simulink model "Simulink_crane_hardware_model_SingleContr_R2016a"  (R2016a)
settings: Solver=ode5  StartTime=0.0  StopTime=inf  FixedStep=1/100  RelTol=1e-3  AbsTol=1e-6
values from neighbouring files (symbols this model uses):
  DTraj = 0.3    [RunHWModel.m]
  ITraj = 0.3    [RunHWModel.m]
  PTraj = 3.0    (= 3)    [RunHWModel.m]
  Ts = 1/20    (= 0.05)    [setup.m]
  waypoints = [waypoints, find_nearest_obstacles(waypoints, Grid)]    [path_planning.m]    (also in path_to_waypoints.m = [])
undefined symbols (not defined in the file or in its folder): Crane3D_RangeBit, Crane3D_ScaleCoeff, xRange, yRange
undefined symbols (not defined in the file): RTDAC4PCIBaseAddress
libraries: simulink x2
(part 11 of 11)

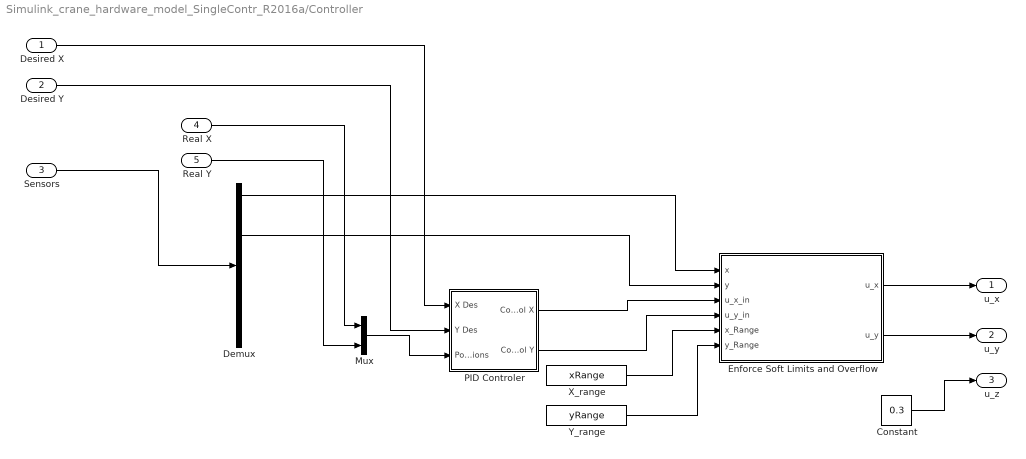
== system Simulink_crane_hardware_model_SingleContr_R2016a/Controller ==
  Desired X : Inport
  Desired Y : Inport  Port=2
  Sensors : Inport  Port=3
  Real X : Inport  Port=4
  Real Y : Inport  Port=5
  Constant : Constant  Value=0.3
  Demux : Demux  Outputs=8
  Enforce Soft Limits and Overflow : MATLAB Function  TreatAsAtomicUnit=on
      settings: PermitHierarchicalResolution=ParametersOnly
  Mux : Mux  Inputs=2
  PID Controler : Subsystem
  X_range : Constant  Value=xRange
  "Y_range " : Constant  Value=yRange
  u_x : Outport
  u_y : Outport  Port=2
  u_z : Outport  Port=3
  wires:
  Constant/1 -> u_z/1
  "Y_range "/1 -> Enforce Soft Limits and Overflow/6(y_Range)
  X_range/1 -> Enforce Soft Limits and Overflow/5(x_Range)
  PID Controler/2(Control Y) -> Enforce Soft Limits and Overflow/4(u_y_in)
  PID Controler/1(Control X) -> Enforce Soft Limits and Overflow/3(u_x_in)
  Desired X/1 -> PID Controler/1(X Des)
  Enforce Soft Limits and Overflow/2(u_y) -> u_y/1
  Enforce Soft Limits and Overflow/1(u_x) -> u_x/1
  Desired Y/1 -> PID Controler/2(Y Des)
  Mux/1 -> PID Controler/3(Positions)
  Sensors/1 -> Demux/1
  Demux/1 -> Enforce Soft Limits and Overflow/1(x)
  Demux/3 -> Enforce Soft Limits and Overflow/2(y)
  Real X/1 -> Mux/1
  Real Y/1 -> Mux/2

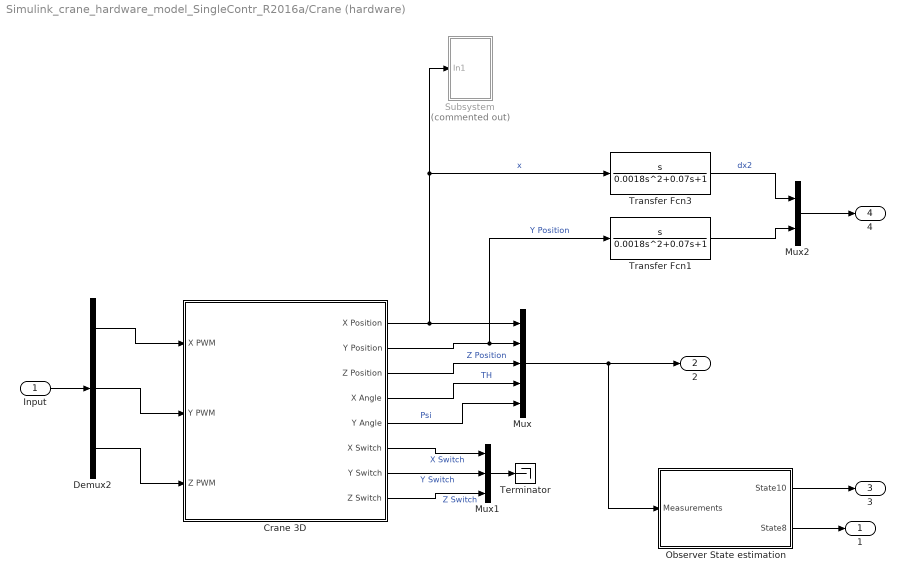
== system Simulink_crane_hardware_model_SingleContr_R2016a/Crane (hardware) ==
  Input : Inport
  Crane 3D : Subsystem  mask{BaseAddress=RTDAC4PCIBaseAddress, T0=1/100}
      mask prompts: BaseAddress "Base Address:"; T0 "Sampling Period:"
      mask Display: image(imread('crane.jpeg'))
  Demux2 : Demux  Outputs=3
  Mux : Mux  Inputs=5
  Mux1 : Mux  Inputs=3
  Mux2 : Mux  Inputs=2
  Observer State estimation : Subsystem
  Subsystem : Subsystem  Commented=on
  Terminator : Terminator
  Transfer Fcn1 : TransferFcn  Numerator=[1 0]  Denominator=[0.0018 0.07 1]
  Transfer Fcn3 : TransferFcn  Numerator=[1 0]  Denominator=[0.0018 0.07 1]
  1 : Outport
  2 : Outport  Port=2
  3 : Outport  Port=3
  4 : Outport  Port=4
  wires:
  Input/1 -> Demux2/1
  Crane 3D/2(Y Position) -> Transfer Fcn1/1, Mux/2  "Y Position"
  Crane 3D/3(Z Position) -> Mux/3  "Z Position"
  Crane 3D/4(X Angle) -> Mux/4  "TH"
  Crane 3D/5(Y Angle) -> Mux/5  "Psi"
  Mux/1 -> 2/1, Observer State estimation/1(Measurements)
  Crane 3D/6(X Switch) -> Mux1/1  "X Switch"
  Crane 3D/7(Y Switch) -> Mux1/2  "Y Switch"
  Crane 3D/8(Z Switch) -> Mux1/3  "Z Switch"
  Demux2/1 -> Crane 3D/1(X PWM)
  Demux2/2 -> Crane 3D/2(Y PWM)
  Demux2/3 -> Crane 3D/3(Z PWM)
  Observer State estimation/2(State8) -> 1/1
  Mux1/1 -> Terminator/1
  Observer State estimation/1(State10) -> 3/1
  Crane 3D/1(X Position) -> Subsystem/1(In1), Transfer Fcn3/1, Mux/1  "x"
  Transfer Fcn3/1 -> Mux2/1  "dx2"
  Transfer Fcn1/1 -> Mux2/2
  Mux2/1 -> 4/1

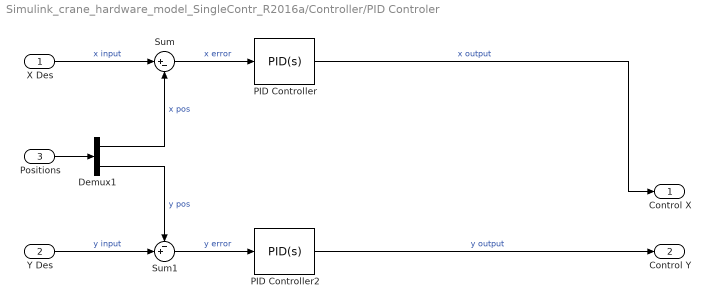
== system Simulink_crane_hardware_model_SingleContr_R2016a/Controller/PID Controler ==
  X Des : Inport
  Y Des : Inport  Port=2
  Positions : Inport  Port=3
  Demux1 : Demux  Outputs=2
  PID Controller : simulink/Continuous/PID Controller  Controller=PID  TimeDomain=Continuous-time  SampleTime=-1  IntegratorMethod=Forward Euler  FilterMethod=Forward Euler  Form=Parallel  UseFilter=on  ControllerParametersSource=internal  P=PTraj  I=ITraj  D=DTraj  N=30  InitialConditionSource=internal  InitialConditionForIntegrator=0  InitialConditionForFilter=0  ExternalReset=none  LimitOutput=on  UpperSaturationLimit=1  LowerSaturationLimit=-1  LinearizeAsGain=on  AntiWindupMode=none  Kb=1  TrackingMode=off  Kt=1  PParamMin=[]  PParamMax=[]  IParamMin=[]  IParamMax=[]  DParamMin=[]  DParamMax=[]  NParamMin=[]  NParamMax=[]  KbParamMin=[]  KbParamMax=[]  KtParamMin=[]  KtParamMax=[]  POutMin=[]  POutMax=[]  IOutMin=[]  IOutMax=[]  DOutMin=[]  DOutMax=[]  NOutMin=[]  NOutMax=[]  KbOutMin=[]  KbOutMax=[]  KtOutMin=[]  KtOutMax=[]  IntegratorOutMin=[]  IntegratorOutMax=[]  FilterOutMin=[]  FilterOutMax=[]  SumOutMin=[]  SumOutMax=[]  SumI1OutMin=[]  SumI1OutMax=[]  SumI2OutMin=[]  SumI2OutMax=[]  SumI3OutMin=[]  SumI3OutMax=[]  SumDOutMin=[]  SumDOutMax=[]  SaturationOutMin=[]  SaturationOutMax=[]  IntegratorContinuousStateAttributes=''  IntegratorStateMustResolveToSignalObject=off  IntegratorRTWStateStorageClass=Auto  FilterContinuousStateAttributes=''  FilterStateMustResolveToSignalObject=off  FilterRTWStateStorageClass=Auto  DifferentiatorICPrevScaledInput=0  DifferentiatorOutMin=[]  DifferentiatorOutMax=[]
  PID Controller2 : simulink/Continuous/PID Controller  Controller=PID  TimeDomain=Continuous-time  SampleTime=-1  IntegratorMethod=Forward Euler  FilterMethod=Forward Euler  Form=Parallel  UseFilter=on  ControllerParametersSource=internal  P=PTraj  I=ITraj  D=DTraj  N=30  InitialConditionSource=internal  InitialConditionForIntegrator=0  InitialConditionForFilter=0  ExternalReset=none  LimitOutput=on  UpperSaturationLimit=1  LowerSaturationLimit=-1  LinearizeAsGain=on  AntiWindupMode=none  Kb=1  TrackingMode=off  Kt=1  PParamMin=[]  PParamMax=[]  IParamMin=[]  IParamMax=[]  DParamMin=[]  DParamMax=[]  NParamMin=[]  NParamMax=[]  KbParamMin=[]  KbParamMax=[]  KtParamMin=[]  KtParamMax=[]  POutMin=[]  POutMax=[]  IOutMin=[]  IOutMax=[]  DOutMin=[]  DOutMax=[]  NOutMin=[]  NOutMax=[]  KbOutMin=[]  KbOutMax=[]  KtOutMin=[]  KtOutMax=[]  IntegratorOutMin=[]  IntegratorOutMax=[]  FilterOutMin=[]  FilterOutMax=[]  SumOutMin=[]  SumOutMax=[]  SumI1OutMin=[]  SumI1OutMax=[]  SumI2OutMin=[]  SumI2OutMax=[]  SumI3OutMin=[]  SumI3OutMax=[]  SumDOutMin=[]  SumDOutMax=[]  SaturationOutMin=[]  SaturationOutMax=[]  IntegratorContinuousStateAttributes=''  IntegratorStateMustResolveToSignalObject=off  IntegratorRTWStateStorageClass=Auto  FilterContinuousStateAttributes=''  FilterStateMustResolveToSignalObject=off  FilterRTWStateStorageClass=Auto  DifferentiatorICPrevScaledInput=0  DifferentiatorOutMin=[]  DifferentiatorOutMax=[]
  Sum : Sum  Inputs=|+-
  Sum1 : Sum  Inputs=-+|
  Control X : Outport
  Control Y : Outport  Port=2
  wires:
  Demux1/1 -> Sum/2  "x pos"
  X Des/1 -> Sum/1  "x input"
  Sum/1 -> PID Controller/1  "x error"
  Sum1/1 -> PID Controller2/1  "y error"
  Demux1/2 -> Sum1/1  "y pos"
  Y Des/1 -> Sum1/2  "y input"
  Positions/1 -> Demux1/1
  PID Controller/1 -> Control X/1  "x output"
  PID Controller2/1 -> Control Y/1  "y output"

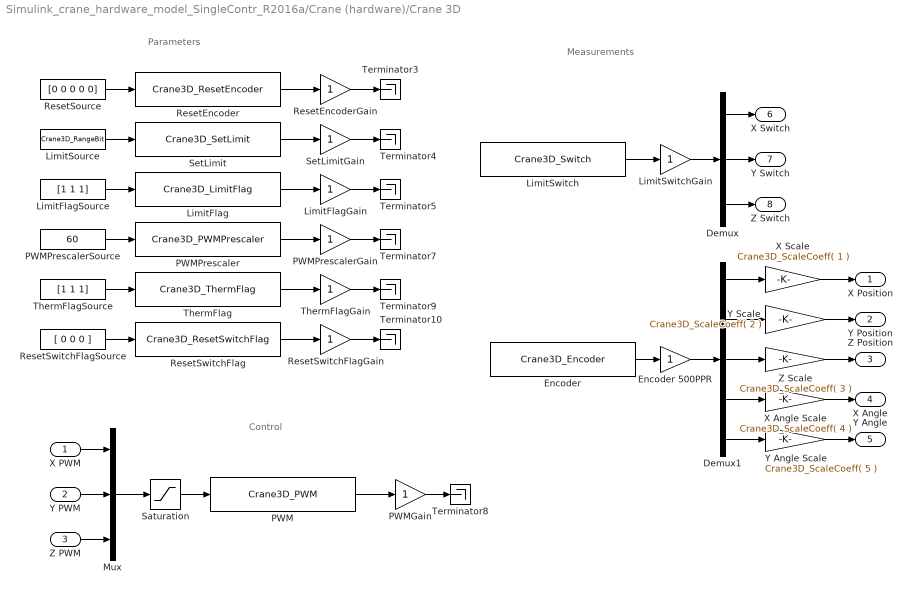
== system Simulink_crane_hardware_model_SingleContr_R2016a/Crane (hardware)/Crane 3D ==
  note: Parameters
  note: Control
  note: Measurements
  X PWM : Inport
  Y PWM : Inport  Port=2
  Z PWM : Inport  Port=3
  Demux : Demux  Outputs=3
  Demux1 : Demux  Outputs=5
  Encoder : S-Function  FunctionName=Crane3D_Encoder  Parameters=BaseAddress, T0  SFunctionDeploymentMode=off  EnableBusSupport=off
  Encoder 500PPR : Gain  SaturateOnIntegerOverflow=on  OutDataTypeStr=Inherit: Same as input  ParamDataTypeStr=Inherit: Same as input
  LimitFlag : S-Function  FunctionName=Crane3D_LimitFlag  Parameters=BaseAddress, T0  SFunctionDeploymentMode=off  EnableBusSupport=off
  LimitFlagGain : Gain  SaturateOnIntegerOverflow=on  OutDataTypeStr=Inherit: Same as input  ParamDataTypeStr=Inherit: Same as input
  LimitFlagSource : Constant  Value=[1 1 1]
  LimitSource : Constant  Value=Crane3D_RangeBit
  LimitSwitch : S-Function  FunctionName=Crane3D_Switch  Parameters=BaseAddress, T0  SFunctionDeploymentMode=off  EnableBusSupport=off
  LimitSwitchGain : Gain  SaturateOnIntegerOverflow=on  OutDataTypeStr=Inherit: Same as input  ParamDataTypeStr=Inherit: Same as input
  Mux : Mux  Inputs=3
  PWM : S-Function  FunctionName=Crane3D_PWM  Parameters=BaseAddress, T0  SFunctionDeploymentMode=off  EnableBusSupport=off
  PWMGain : Gain  SaturateOnIntegerOverflow=on  OutDataTypeStr=Inherit: Same as input  ParamDataTypeStr=Inherit: Same as input
  PWMPrescaler : S-Function  FunctionName=Crane3D_PWMPrescaler  Parameters=BaseAddress, T0  SFunctionDeploymentMode=off  EnableBusSupport=off
  PWMPrescalerGain : Gain  SaturateOnIntegerOverflow=on  OutDataTypeStr=Inherit: Same as input  ParamDataTypeStr=Inherit: Same as input
  PWMPrescalerSource : Constant  Value=60
  ResetEncoder : S-Function  FunctionName=Crane3D_ResetEncoder  Parameters=BaseAddress, T0  SFunctionDeploymentMode=off  EnableBusSupport=off
  ResetEncoderGain : Gain  SaturateOnIntegerOverflow=on  OutDataTypeStr=Inherit: Same as input  ParamDataTypeStr=Inherit: Same as input
  ResetSource : Constant  Value=[0 0 0 0 0]
  "ResetSwitchFlag " : S-Function  FunctionName=Crane3D_ResetSwitchFlag  Parameters=BaseAddress, T0  SFunctionDeploymentMode=off  EnableBusSupport=off
  ResetSwitchFlagGain : Gain  SaturateOnIntegerOverflow=on  OutDataTypeStr=Inherit: Same as input  ParamDataTypeStr=Inherit: Same as input
  ResetSwitchFlagSource : Constant  Value=[ 0 0 0 ]
  Saturation : Saturate  UpperLimit=1  LowerLimit=-1
  SetLimit : S-Function  FunctionName=Crane3D_SetLimit  Parameters=BaseAddress, T0  SFunctionDeploymentMode=off  EnableBusSupport=off
  SetLimitGain : Gain  SaturateOnIntegerOverflow=on  OutDataTypeStr=Inherit: Same as input  ParamDataTypeStr=Inherit: Same as input
  Terminator{3..5,7..10} (7 alike) : Terminator
  "ThermFlag " : S-Function  FunctionName=Crane3D_ThermFlag  Parameters=BaseAddress, T0  SFunctionDeploymentMode=off  EnableBusSupport=off
  ThermFlagGain : Gain  SaturateOnIntegerOverflow=on  OutDataTypeStr=Inherit: Same as input  ParamDataTypeStr=Inherit: Same as input
  ThermFlagSource : Constant  Value=[1 1 1]
  X Angle Scale : Gain  Gain=Crane3D_ScaleCoeff( 4 )  OutDataTypeStr=Inherit: Same as input  ParamDataTypeStr=Inherit: Same as input
  X Scale : Gain  Gain=Crane3D_ScaleCoeff( 1 )  OutDataTypeStr=Inherit: Same as input  ParamDataTypeStr=Inherit: Same as input
  Y Angle Scale : Gain  Gain=Crane3D_ScaleCoeff( 5 )  OutDataTypeStr=Inherit: Same as input  ParamDataTypeStr=Inherit: Same as input
  Y Scale : Gain  Gain=Crane3D_ScaleCoeff( 2 )  OutDataTypeStr=Inherit: Same as input  ParamDataTypeStr=Inherit: Same as input
  Z Scale : Gain  Gain=Crane3D_ScaleCoeff( 3 )  OutDataTypeStr=Inherit: Same as input  ParamDataTypeStr=Inherit: Same as input
  X Position : Outport  InitialOutput=0
  Y Position : Outport  Port=2  InitialOutput=0
  Z Position : Outport  Port=3  InitialOutput=0
  X Angle : Outport  Port=4  InitialOutput=0
  Y Angle : Outport  Port=5  InitialOutput=0
  X Switch : Outport  Port=6  InitialOutput=0
  Y Switch : Outport  Port=7  InitialOutput=0
  Z Switch : Outport  Port=8  InitialOutput=0
  wires:
  Encoder 500PPR/1 -> Demux1/1
  Encoder/1 -> Encoder 500PPR/1
  Saturation/1 -> PWM/1
  Mux/1 -> Saturation/1
  PWM/1 -> PWMGain/1
  PWMGain/1 -> Terminator8/1
  ResetEncoder/1 -> ResetEncoderGain/1
  SetLimit/1 -> SetLimitGain/1
  LimitFlag/1 -> LimitFlagGain/1
  PWMPrescaler/1 -> PWMPrescalerGain/1
  "ThermFlag "/1 -> ThermFlagGain/1
  "ResetSwitchFlag "/1 -> ResetSwitchFlagGain/1
  ResetSource/1 -> ResetEncoder/1
  LimitSource/1 -> SetLimit/1
  LimitFlagSource/1 -> LimitFlag/1
  PWMPrescalerSource/1 -> PWMPrescaler/1
  ThermFlagSource/1 -> "ThermFlag "/1
  ResetSwitchFlagSource/1 -> "ResetSwitchFlag "/1
  ResetEncoderGain/1 -> Terminator3/1
  SetLimitGain/1 -> Terminator4/1
  LimitFlagGain/1 -> Terminator5/1
  PWMPrescalerGain/1 -> Terminator7/1
  ThermFlagGain/1 -> Terminator9/1
  ResetSwitchFlagGain/1 -> Terminator10/1
  Z PWM/1 -> Mux/3
  Y PWM/1 -> Mux/2
  X PWM/1 -> Mux/1
  LimitSwitch/1 -> LimitSwitchGain/1
  LimitSwitchGain/1 -> Demux/1
  Demux/1 -> X Switch/1
  Demux/2 -> Y Switch/1
  Demux/3 -> Z Switch/1
  Z Scale/1 -> Z Position/1
  X Scale/1 -> X Position/1
  Y Scale/1 -> Y Position/1
  Y Angle Scale/1 -> Y Angle/1
  X Angle Scale/1 -> X Angle/1
  Demux1/5 -> Y Angle Scale/1
  Demux1/4 -> X Angle Scale/1
  Demux1/3 -> Z Scale/1
  Demux1/2 -> Y Scale/1
  Demux1/1 -> X Scale/1

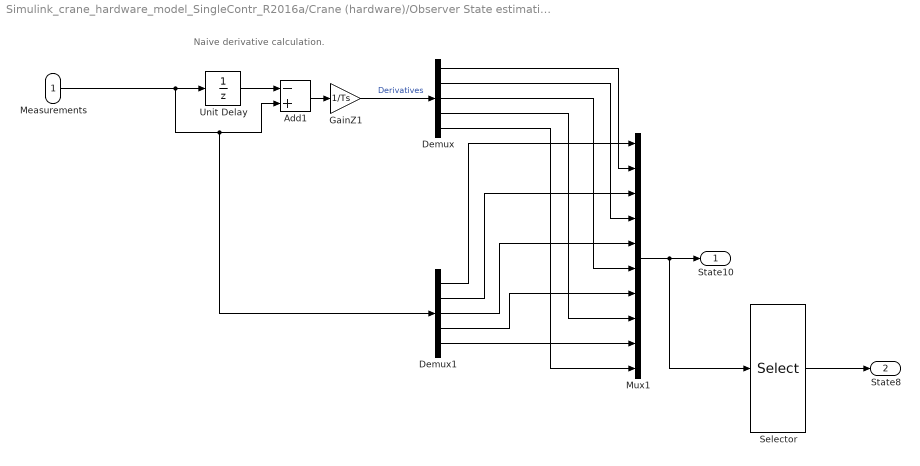
== system Simulink_crane_hardware_model_SingleContr_R2016a/Crane (hardware)/Observer State estimation ==
  note: Naive derivative calculation.
  Measurements : Inport
  Add1 : Sum  Inputs=-+
  Demux : Demux  Outputs=5
  Demux1 : Demux  Outputs=5
  GainZ1 : Gain  Gain=1/Ts  SaturateOnIntegerOverflow=on  OutDataTypeStr=Inherit: Same as input  ParamDataTypeStr=Inherit: Same as input
  Mux1 : Mux  Inputs=10
  Selector : Selector  InputPortWidth=10  IndexOptions=Index vector (dialog)  Indices=[1:4 7:10]  OutputSizes=1
  Unit Delay : UnitDelay  InitialCondition="[0.26 0.32 0.3  0 0]"  SampleTime=-1
  State10 : Outport
  State8 : Outport  Port=2
  wires:
  Unit Delay/1 -> Add1/1
  Add1/1 -> GainZ1/1
  Measurements/1 -> Demux1/1, Add1/2, Unit Delay/1
  GainZ1/1 -> Demux/1  "Derivatives"
  Mux1/1 -> Selector/1, State10/1
  Demux1/1 -> Mux1/1
  Demux/1 -> Mux1/2
  Demux1/2 -> Mux1/3
  Demux1/3 -> Mux1/5
  Demux1/4 -> Mux1/7
  Demux1/5 -> Mux1/9
  Demux/2 -> Mux1/4
  Demux/3 -> Mux1/6
  Demux/4 -> Mux1/8
  Demux/5 -> Mux1/10
  Selector/1 -> State8/1

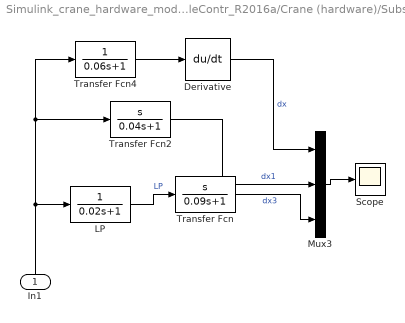
== system Simulink_crane_hardware_model_SingleContr_R2016a/Crane (hardware)/Subsystem ==
  In1 : Inport
  Derivative : Derivative
  LP : TransferFcn  Numerator=[0 1]  Denominator=[0.02 1]
  Mux3 : Mux  Inputs=3
  Scope : Scope
  Transfer Fcn : TransferFcn  Numerator=[1 0]  Denominator=[0.09 1]
  Transfer Fcn2 : TransferFcn  Numerator=[1 0]  Denominator=[0.04 1]
  Transfer Fcn4 : TransferFcn  Numerator=[0 1]  Denominator=[0.06 1]
  wires:
  LP/1 -> Transfer Fcn/1  "LP"
  Transfer Fcn2/1 -> Mux3/2  "dx1"
  Transfer Fcn4/1 -> Derivative/1
  Transfer Fcn/1 -> Mux3/3  "dx3"
  Derivative/1 -> Mux3/1  "dx"
  Mux3/1 -> Scope/1
  In1/1 -> Transfer Fcn4/1, Transfer Fcn2/1, LP/1

== matlab function Simulink_crane_hardware_model_SingleContr_R2016a/Controller/Enforce Soft Limits and Overflow ==
  data: x input; u_x output; y input; u_x_in input; u_y_in input; x_Range input; y_Range input; u_y output
function [u_x, u_y] = fcn(x, y, u_x_in, u_y_in, x_Range, y_Range)

buff_up = 0.08;
buff_low = 0.08;
u_x = u_x_in;
u_y = u_y_in;

% Deal with overflow - may not be the most appropriate place
if(x > 10 || x < -10)
   x = 0;
end
if (y > 10 || y < -10)
   y = 0;
end

% Put in place soft boundaries on the borders
if (x > (x_Range(2)-buff_up))
    u_x = min(u_x_in,0);
end

if (x < (x_Range(1)+buff_low))
    u_x = max(u_x_in,0);
end


if (y > (y_Range(2)-buff_up))
    u_y = min(u_y_in,0);
end

if (y < (y_Range(1)+buff_low))
    u_y = max(u_y_in,0);
end


end

== matlab function Simulink_crane_hardware_model_SingleContr_R2016a/Select most convenient path ==
  data: x output; y output; x_pos input; y_pos input; Waypoints input
function [x,y] = Path_Selector(x_pos, y_pos, Waypoints)
persistent WP_Index

if isempty(WP_Index)
    WP_Index = 1;
end
    
x = Waypoints(WP_Index,1)/100;
y = Waypoints(WP_Index,2)/100;
x_max = x+0.015;
x_min = x-0.015;
y_max = y+0.015;
y_min = y-0.015;

%% Crane arrived to point
if (((x_pos <= x_max) && (x_pos >= x_min)) && ((y_pos <= y_max) && (y_pos >= y_min)))
    WP_Index = WP_Index + 1; 
    if WP_Index > (size(Waypoints))
        WP_Index = WP_Index - 1;
    end
end

== matlab function Simulink_crane_hardware_model_SingleContr_R2016a/Convert Coordinates ==
  data: x output; y output; Sensors input
function [x,y] = Sensors2World(Sensors)

%% Assumptions
R = 0.3;

%% Obtain Measurements from sensors
now_x = Sensors(1);
now_y = Sensors(3);
now_alpha = Sensors (7) + pi/2;
now_beta = Sensors(5);

sin_a = sin(now_alpha);
sin_b = sin(now_beta);
cos_a = cos(now_alpha);

x = now_x + R * sin_a * sin_b;
y = now_y + R * cos_a;
